simulink model "simulink_act1_ses1_grupo1_exp1"  (R2021b)
settings: Solver=ode1  StartTime=0.0  StopTime=10.0  FixedStep=0.1  RelTol=1e-3
settings Model: Creator=LABCONTROL1  LastModifiedBy=LABCONTROL1

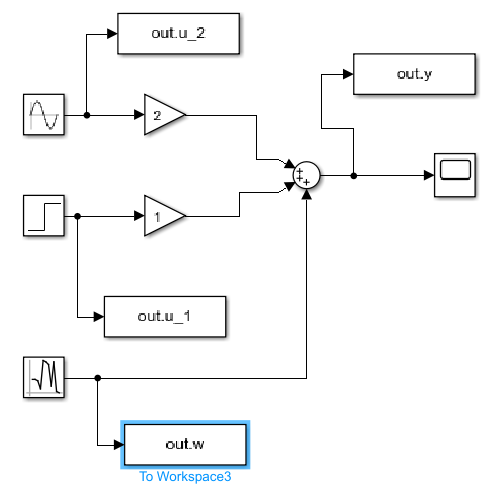
[thumbnail: Simulink's stored preview of the top-level diagram]
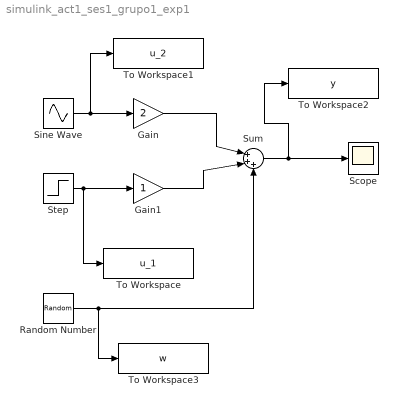
== system simulink_act1_ses1_grupo1_exp1 ==
  Gain : Gain  Gain=2
  Gain1 : Gain
  Random Number : RandomNumber  Variance=0.1  SampleTime=0.1
  Scope : Scope
  Sine Wave : Sin  Frequency=10  SampleTime=0
  Step : Step  SampleTime=0
  Sum : Sum  Inputs=|+++
  To Workspace : ToWorkspace  VariableName=u_1  SampleTime=0.5
      settings: Save2DSignal=2-D array (concatenate along first dimension)
  To Workspace1 : ToWorkspace  VariableName=u_2  SampleTime=0.5
      settings: Save2DSignal=2-D array (concatenate along first dimension)
  To Workspace2 : ToWorkspace  VariableName=y  SampleTime=0.5
      settings: Save2DSignal=2-D array (concatenate along first dimension)
  To Workspace3 : ToWorkspace  VariableName=w  SampleTime=0.5
      settings: Save2DSignal=2-D array (concatenate along first dimension)
  wires:
  Sine Wave/1 -> To Workspace1/1, Gain/1
  Gain/1 -> Sum/1
  Gain1/1 -> Sum/2
  Step/1 -> To Workspace/1, Gain1/1
  Random Number/1 -> To Workspace3/1, Sum/3
  Sum/1 -> To Workspace2/1, Scope/1
